simulink model "Demo_AU_VA"  (R2014a)
settings: Solver=FixedStepDiscrete  StartTime=0.0  StopTime=inf  FixedStep=0.01  RelTol=1e-3
undefined symbols (not defined in the file or in its folder): clock, lib_affectiveChar_behavior, notImitateSmile, Stateflow
libraries: simulink x6, realtime_pacer_lib x2
(part 2 of 2)

== stateflow chart Demo_AU_VA/facialExpr/facialExpression_Controller ==
  state subFaceTwitch [parallel]
    settings: executionOrder=3
    state init
      entry:
      num=randi([1,100]);
    state randFace
      entry:
      randNum=randi([1,2]);
      [pp,BMLl]=faceTwitch(randNum);
      newBmlsL=insertQueueLow(bmlsL,BMLl); bmlsL=newBmlsL;
    init -> randFace [order 1] : [num>100]
    randFace -> init : after(3,secs)
    (default) -> init
    init -> init [order 2] : after(5,secs)
  state subFacial [parallel]
    settings: executionOrder=1
    state stateFacialExpression
      entry:
      emotion_amount_factor =set_AU_Amount(inA,inV);
      BMLl=cmdBML_AU_VA(emotion_amount_factor);
      newBmlsL=insertQueueLow(bmlsL,BMLl); bmlsL=newBmlsL;
    state initial
    state wait
    (default) -> subFacial.initial
    subFacial.initial -> subFacial.stateFacialExpression : [inA==-1000]
    wait -> subFacial.stateFacialExpression : after(7,secs)
    subFacial.stateFacialExpression -> wait
  state subFacial1 [parallel]
    settings: executionOrder=2
    state stateFacialExpression
      entry:[au,au_L]=setAU(internalE);
      emotion_amount_factor2 =set_eAmountFactor(internalE,au,inA,inV);
      BMLl=cmdBML_AUmerg(au,emotion_amount_factor2,au_L);
      newBmlsL=insertQueueLow(bmlsL,BMLl); bmlsL=newBmlsL;
    state initial
      entry:
      au=[0,0,0,0,0,0];
      au_L=0;
    state wait3
    (default) -> subFacial1.initial
    subFacial1.initial -> subFacial1.stateFacialExpression
    wait3 -> subFacial1.stateFacialExpression : after(7,secs)
    subFacial1.stateFacialExpression -> wait3
  data: p function_output double size=1; bmlID function_input double; poseBML function_output double size=[1000,1]; eAmountFactor function_output double size=[1,11]; arousal function_input double size=1; valence function_input double size=1; bmls function_input double size=[1000,5]; myBML function_input double size=[1000,1]; newBmls function_output double size=[1000,5]; E function_input double size=1; AU function_output double size=[1,6]; L function_output double size=1; E function_input double size=1; eAmountFactor2 function_output double size=[1,6]; AU function_input double size=[1,6]; arousal function_input double size=1; valence function_input double size=1; bmlsL data_store_memory size=[256,1]; BMLl local double size=[1000,1]; newBmlsL local double size=[1000,5]; inA input double size=1; inV input double size=1; emotion_amount_factor output double size=[1,11]; internalE input double size=1; emotion_amount_factor2 output double size=[1,6]; au_L local; au local; randTwitch input double size=1; randNum local; pp local; num local
  events: secs input RISING_EDGE_EVENT
  function [p,poseBML] = faceTwitch(bmlID):
    | function [p,poseBML] = faceTwitch(bmlID)
    | 
    | aVarTruthTableCondition_1 = false;
    | aVarTruthTableCondition_2 = false;
    | 
    | 
    | % brow
    | 
    | aVarTruthTableCondition_1 = logical(bmlID==1);
    | 
    | % fear
    | 
    | aVarTruthTableCondition_2 = logical(bmlID==2);
    | 
    | if (aVarTruthTableCondition_1)
    |     aFcnTruthTableAction_1();
    | elseif (aVarTruthTableCondition_2)
    |     aFcnTruthTableAction_2();
    | else % Default
    |     aFcnTruthTableAction_2();
    | end
    | 
    | function aFcnTruthTableAction_1()
    | 
    | % faceTwitch
    | 
    | poseBML=encStr2Arr('<?xml version="1.0" ?><act><bml><face amount="0.5" au="1" start="0" end="0.5" side="BOTH" type="facs"/><face amount="1" au="2"  start="0" end="0.5"  side="BOTH"  type="facs"/><face amount="0.5"  start="0" end="0.5"  au="5" side="BOTH" type="facs"/></bml></act>');p=3;
    | 
    | function aFcnTruthTableAction_2()
    | 
    | % fear
    | 
    | poseBML=encStr2Arr('<?xml version="1.0" ?><act><bml><face amount="0.3" au="1" end="4" ready="1" relax="3" side="BOTH" start="0" stroke="2" type="facs"/><face amount="0.5" au="5" end="4" ready="1" relax="3" side="BOTH" start="0" stroke="2" type="facs"/></bml></act>');p=3;
  function eAmountFactor =set_AU_Amount(arousal,valence):
    | function eAmountFactor =set_AU_Amount(arousal,valence)
    |     %15-12-2015, PAD drivern facial expr simul, Grammer data to map AU and VA
    | %     fprintf('VA: %0.0f,%0.0f\r\n',arousal,valence);
    |     %scale
    | %     p = valence * (20/9)  - 10;
    | %     a = arousal * (20/9)  - 10;
    | 
    |     p=valence;a=arousal;
    |    all_AUs=[1,2,4,5,6,7,12,26,45,10,25];eAmountFactor=[0,0,0,0,0,0,0,0,0,0,0];
    |     for c=1:12
    |         eAmountFactor(1)=(0.003*p-0.002*a)*1.2;  %1,inner 
    |         eAmountFactor(2)=-0.002*p + 0.010*a; %2
    | %         eAmountFactor(12)=-0.016*p+0.034*a; %26
    |         eAmountFactor(8)=-0.002*p+0.023*a;  %26,-0.002*p+0.049*a
    |         eAmountFactor(5)=-0.008*p+0.009*a;  %6
    |     %   eAmountFactor=0.002*p+0.004*a;  %18 lip Puckerer, W 0.3
    |     %   eAmountFactor=0.007*p+0.025*a;  %22 lip fumeler, ShCh 0.5
    |     %   eAmountFactor=0.003*p+0.009*a; %14 dimpler FV+PBM 0.5
    |     %   eAmountFactor=-0.010*p+0.017*a %17 chin raiser
    |         eAmountFactor(10)=-0.020*p+0.020*a;  %10 upper lip raiser,-0.053*p+0.026*a
    |         eAmountFactor(4)=-0.003*p+0.032*a; %5 upper lid raiser
    |         eAmountFactor(9)=-0.011*p-0.011*a; %eye closed, 45 instead of 43,-0.021*p-0.037*a
    |         eAmountFactor(3)=-0.036*p+0.022*a; %4 brow lowerer
    |     %   eAmountFactor=-0.008*p+0.006*a;    %9 nose wrikler ,10
    |     %   eAmountFactor=-0.004*p+0.004*a;    %39?
    |     %   eAmountFactor=-0.010*p+0.008*a;    %38?
    |         eAmountFactor(11)=-0.011*p+0.023*a;%25 lip open,-0.023*p+0.058*a
    |     %   eAmountFactor=-0.004*p-0.003*a;    %24 lip pressor, PBM 
    |     %   eAmountFactor=-0.011*p+0.009*a;    %23 lip tightner PBM0.2 + W0.6
    |     %   eAmountFactor=-0.004*p+0.003*a;    %19?
    |     %   eAmountFactor(8)=0.039*p+0.015*a;  %13 cheek puffer, W 0.3
    |         eAmountFactor(6)=-0.005*p-0.001*a; %7  Lid Tightener
    |         eAmountFactor(7)=0.057*p+0.009*a;  %12 Lip Corner Puller
    |     %   eAmountFactor=-0.008*p+0.009*a;    %11 Nasolabial Deepener
    |     %   eAmountFactor=-0.046*p-0.002*a;    %15 Lip Corner Depressor
    |     %   eAmountFactor=-0.014*p+0.016*a;    %16 Lower Lip Depressor
    |     %   eAmountFactor(20)=-0.026*p+0.010*a;%20 lip stretch
    |         
    |         eAmountFactor=eAmountFactor/6; %scale
    |         
    |     end
  function newBmls =insertQueueLow(bmls,myBML):
    | function newBmls =insertQueueLow(bmls,myBML)
    |     full=1;
    |     t=encStr2Arr(' ');
    |     newBmls=[t t t t t];
    |     for i = 1:5
    |         if (isequal(bmls(:,i),t))
    |             %add to end of the queue where its empty
    |             bmls(:,i)=myBML;
    |             full=0;
    |             break
    |         end
    |     end
    |     if(full~=0)
    |             %if queue full, shift all elements to left which removes the first one, then add to end
    |             bmls(:,1)= bmls(:,2);
    |             bmls(:,2)= bmls(:,3);
    |             bmls(:,3)= bmls(:,4);
    |             bmls(:,5)=myBML;
    |     end
    |     newBmls=bmls;
  function [AU,L]=setAU(E):
    | function [AU,L]=setAU(E)	
    | % 1	Inner Brow Raiser,% 2	Outer Brow Raiser, % 4	Brow Lowerer
    | % 5	Upper Lid Raiser,% 6	Cheek Raiser,% 7	Lid Tightener
    | % 8	Lips Toward Each Other,% 9	Nose Wrinkler,% 10	Upper Lip Raiser	
    | % 11	Nasolabial Deepener	% 12	Lip Corner Puller % 13	Sharp Lip Puller % 14	Dimpler	
    | % 15	Lip Corner Depressor % 16	Lower Lip Depressor % 17	Chin Raiser	mentalis
    | % 18	Lip Pucker	% 19	Tongue Show	% 20	Lip Stretcher % 21	Neck Tightener	platysma
    | % 22	Lip Funneler% 23	Lip Tightener% 24	Lip Pressor % 25	Lips Part	depressor
    | % 26	Jaw Drop,% 27	Mouth Stretch
    | % 43	Eyes Closed, % 44	Eyebrow Gatherer,% 45	Blink,% 46	Wink
    | %smartbody no 43,15,17,10 looks wierd,no 142
    |    AU=[0,0,0,0,0,0];L=0;
    |    % AU5(eyeOpen) for A+
    |    % AU1,4 for V-
    |    %AU12 for V+
    |     switch(E)
    |         case 1 %V- A-,bored (43)[1]
    |             AU=[1,2,45,0,0,0];L=3;%[1,1,0.35]
    |         
    |         case 2 %V- A-;sad %(1,2,4,10,15,17,43)[];can be [1,2,4,45,6,0]
    |             AU=[1,4,0,0,0,0];L=2;%[1,1,0,0,0,0]
    |         
    |         case 3 %V- A+,frust(2,1,14)[1],(-1,-2,4,7,14)[2], maybe(1,7)[0.7,0.7,0.5]
    |             AU=[1,2,4,5,6,0];L=5;%[1,1,1,0.5,0.5,0]
    |         
    |         case 4 %V- A+,fear(1,2,4,5,25=mouth)
    |             AU=[1,2,4,5,6,7];L=6; %[1,1,1,0.2,0.2]
    |         
    |         case 5%V+ A-,sleepy
    |             AU=[12,45,0,0,0,0];L=2;%[0.7,0.3,0,0,0,0]
    |         
    |         case 6%V+ A-,pleased
    |             AU=[6,12,0,0,0,0];L=2;%[0.5,0.7,0,0,0,0]
    |             
    |         case 7%V+ A+,happy
    |             AU=[6,12,1,2,0,0];L=4;%[1,0.5,0,0,0,0]
    |         
    |         case 8%V+ A+,excited
    |             AU=[12,26,5,1,2,6];L=6;%[1,1,1,1,1,0]
    |         
    |         case 9%V- A+, angry
    |             AU=[2,4,5,7,45,0];L=5;%[0.5,1,0.2,0.2,0.2]
    |         
    |         otherwise
    |             %confusion (1,2,4,7)[1] %[1,1,1,0.2]
    |             %worried (1,2,4,5) [1,1,1,0.5]
    |             %angry(4,5,7,10,27)[], can be(2,4,5,7,45)[0.5,1,0.2,0.2,0.2]
    | 
    |             AU=[0,0,0,0,0,0];L=0;
    |             disp('error, setAU,emotion not listed');
    |     end  
    | %[1]Craig S.D. et al(2004)emotions during learning:the first steps tw affect sensitive
    | %[2]grafsgard J F () automatically recog facial indicator of frust
  function eAmountFactor2 =set_eAmountFactor(E,AU,arousal,valence):
    | function eAmountFactor2 =set_eAmountFactor(E,AU,arousal,valence)
    | coder.extrinsic('fscanf')
    | coder.extrinsic('get_param');
    |     eAmountFactor2=[0,0,0,0,0,0];pFactor=0.8;    
    |     p=1;
    |     if(p==1)
    |         %HEHN
    |         if(E==1)  %bored [1,2,45]
    |             eAmountFactor2=[1,1,0.25,0,0,0];
    |         elseif(E==2) %sad [1,4]
    |             eAmountFactor2=[0.7,1,0,0,0,0];
    |         elseif(E==3) %frust [1,2,4,5,6]
    |             eAmountFactor2=[1,1,1,0.7,0.7,0];
    |         elseif(E==4) %fear[1,2,4,5,6,7]
    |             eAmountFactor2=[1,1,1,0.8,0.8,0.2];
    |         elseif(E==5)%sleepy[12,45,0,0,0,0]
    |             eAmountFactor2=[0.7,0.25,0,0,0,0];
    |         elseif(E==6)%pleased[6,12,0,0,0,0]
    |             eAmountFactor2=[0.4,0.4,0,0,0,0];    
    |         elseif(E==7)%happy[6,12,0,0,0,0]
    |             eAmountFactor2=[0.9,1.2,0,0,0,0];
    |         elseif(E==8)%excited [12,26,5,1,2,6]
    |             eAmountFactor2=[0.7,0.5,0.8,0.8,0.8,0.5];    
    |         else          
    |             eAmountFactor2=[0,0,0,0,0,0];
    |             disp('error, set_eAmountFactor,emotion not listed');
    |         end
    |         eAmountFactor2=eAmountFactor2;
    |         %LEHN  
    |     elseif(p==2)
    |         if(E==1)  %bored [1,2,45]
    |             eAmountFactor2=[1,1,0.25,0,0,0];
    |         elseif(E==2) %sad [1,4]
    |             eAmountFactor2=[0.7,1,0,0,0,0];
    |         elseif(E==3) %frust [1,2,4,5,6]
    |             eAmountFactor2=[1,1,1,0.7,0.7,0];
    |         elseif(E==4) %fear[1,2,4,5,6,7]
    |             eAmountFactor2=[1,1,1,0.8,0.8,0.2];
    |         elseif(E==5)%sleepy[12,45,0,0,0,0]
    |             eAmountFactor2=[0.7,0.25,0,0,0,0];
    |         elseif(E==6)%pleased[6,12,0,0,0,0]
    |             eAmountFactor2=[0.4,0.4,0,0,0,0];    
    |         elseif(E==7)%happy[6,12,0,0,0,0]
    |             eAmountFactor2=[0.9,1.2,0.4,0.4,0,0];
    |         elseif(E==8)%excited [12,26,5,1,2,0]
    |             eAmountFactor2=[0.7,0.5,0.8,0.8,0.8,0];    
    |         else
    |             eAmountFactor2=[0,0,0,0,0,0];
    |             disp('error, set_eAmountFactor,emotion not listed');
    |         end
    |         eAmountFactor2=eAmountFactor2;
    |         %HELN
    |    elseif(p==3)
    |         if(E==1)  %bored [1,2,45]
    |             eAmountFactor2=[1,1,0.25,0,0,0];
    |         elseif(E==2) %sad [1,4]
    |             eAmountFactor2=[0.7,1,0,0,0,0];
    |         elseif(E==3) %frust [1,2,4,5,6]
    |             eAmountFactor2=[1,1,1,0.7,0.7,0];
    |         elseif(E==4) %fear[1,2,4,5,6,7]
    |             eAmountFactor2=[1,1,1,0.8,0.8,0.2];
    |         elseif(E==5)%sleepy[12,45,0,0,0,0]
    |             eAmountFactor2=[0.7,0.25,0,0,0,0];
    |         elseif(E==6)%pleased[6,12,0,0,0,0]
    |             eAmountFactor2=[0.4,0.4,0,0,0,0];    
    |         elseif(E==7)%happy[6,12,1,2,0,0]
    |             eAmountFactor2=[0.9,1.2,0.4,0.4,0,0];
    |         elseif(E==8)%excited [12,26,5,1,2,0]
    |             eAmountFactor2=[0.7,0.5,0.8,0.8,0.8,0];    
    |         else                    
    |             eAmountFactor2=[0,0,0,0,0,0];
    |             disp('error, set_eAmountFactor,emotion not listed');
    |         end
    |         eAmountFactor2=eAmountFactor2*pFactor;
    |         %LELN
    |     elseif(p==4)
    |          if(E==1)  %bored [1,2,45]
    |             eAmountFactor2=[1,1,0.25,0,0,0];
    |         elseif(E==2) %sad [1,4]
    |             eAmountFactor2=[0.7,1,0,0,0,0];
    |         elseif(E==3) %frust [1,2,4,5,6]
    |             eAmountFactor2=[1,1,1,0.7,0.7,0];
    |         elseif(E==4) %fear[1,2,4,5,6,7]
    |             eAmountFactor2=[1,1,1,0.8,0.8,0.2];
    |         elseif(E==5)%sleepy[12,45,0,0,0,0]
    |             eAmountFactor2=[0.7,0.25,0,0,0,0];
    |         elseif(E==6)%pleased[6,12,0,0,0,0]
    |             eAmountFactor2=[0.4,0.4,0,0,0,0];    
    |         elseif(E==7)%happy[6,12,0,0,0,0]
    |             eAmountFactor2=[0.9,1.2,0.4,0.4,0,0];
    |         elseif(E==8)%excited [12,26,5,1,2,0]
    |             eAmountFactor2=[0.7,0.5,0.8,0.8,0.8,0];    
    |         else                    
    |             eAmountFactor2=[0,0,0,0,0,0];
    |             disp('error, set_eAmountFactor,emotion not listed');
    |         end
    |         eAmountFactor2=eAmountFactor2*pFactor;
    |     end
    |     %7-12-2015: 
    |     % map amount of expressed emotion to valence-arousal value
    |     % valence-arousal change btw 0 and 100; amount changes btw 0.5 and 1
    |     % (values less than 0.4 are not visible)
    |     a_factor=abs(0.4 + arousal/250);
    |     v_factor=abs(0.4 +valence/250);
    | 
    |     % amount of AU 1,2,5,26 changes as a linear function of arousal changes
    |     % amount of AU 4,6,12 changes as a linear function of valence changes
    |     for c = 1:6
    |         if(arousal>0)
    |             if (AU(c)==1|| AU(c)==2|| AU(c)==5|| AU(c)==26)
    |                 eAmountFactor2(c)=eAmountFactor2(c)*a_factor;
    |             end
    |         end
    |         if(valence>0)
    |             if (AU(c)==6|| AU(c)==12)
    |                 eAmountFactor2(c)=eAmountFactor2(c)*v_factor;
    |             end
    |         else% if v<0
    |             if(AU(c)==4)
    |                  eAmountFactor2(c)=eAmountFactor2(c)*v_factor;
    |             end
    |         end    
    |     end
    |     
    | % 10-12-2015
    | % trying to write all the AUs and their amounts in a matrix, failed! 
    | % matlab gives error in writing variable size matrix into a file using fprintf
    | %     All_AUs=[1,2,4,5,6,7,12,26,45];All_AUs_Amounts=[0,0,0,0,0,0,0,0,0];
    | %     for i = 1:9
    | %         t=1;
    | %         for c = 1:6
    | %             if (All_AUs(i)==AU(c))
    | %               All_AUs_Amounts(t,i)= eAmountFactor(c);
    | %               t=t+1;
    | %             end
    | %         end
    | %     end
    | % disp(All_AUs_Amounts)
    | %      fileID = fopen('All_AUs_Amouns_table.txt','a');
    | %      fprintf(fileID,'%s\r\n',All_AUs_Amounts);
    | %      fclose(fileID);
    | 
    | %Following is if we want a same factor for each personaliy all through AUs
    | % function eAmountFactor =set_eAmountFactor(E,P)
    | %     AU=[6,12,142,0,0,0];eAMOUNT=[0,0,0,0,0,0];
    | %     switch E
    | %         case 1  %bored
    | %             eAMOUNT=[1,1,1,0,0,0];
    | %         case 2 %sad
    | %             eAMOUNT=[0.7,0.4,0.9,0,0,0];
    | %         case 3 %angry
    | %             eAMOUNT=[1,0.8,1,0,0,0];
    | %         case 4 %fear
    | %             eAMOUNT=[1,1,1,0,0,0];%5,6,7,26
    | %         case 5%contempt
    | %             eAMOUNT=[1,1,1,0,0,0];
    | %         case 7%happy
    | %             eAMOUNT=[0.2,1,0,0,0,0];
    | %         otherwise           
    | %             eAMOUNT=[0,0,0,0,0,0];
    | %             disp('error,amount for emotion not listed:');disp('eAMOUNT');
    | %     end 
    | %     switch P
    | %         case 1 %HEHN
    | %             pFactor=1;
    | %         case 2 %LEHN
    | %             pFactor=1;
    | %         case 3 %HELN
    | %             pFactor=0.5;
    | %         case 4 %LELN
    | %             pFactor=0.5;
    | %     end
    | %     eAmountFactor=pFactor*eAMOUNT;
